simulink model "heatpump"  (R2021b)
settings: Solver=VariableStepAuto  StartTime=0.0  StopTime=10.0  RelTol=1e-3
settings Model: Creator=Sam  LastModifiedBy=Sam

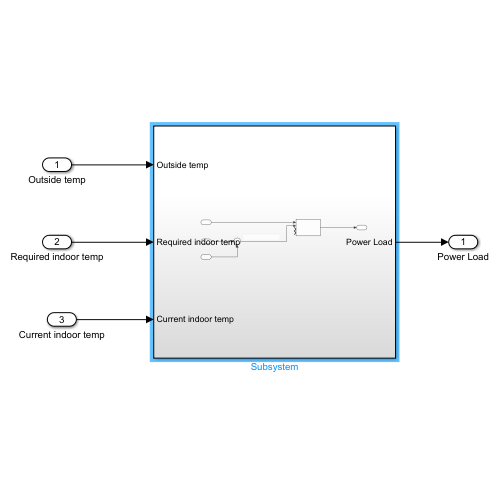
[thumbnail: Simulink's stored preview of the top-level diagram]
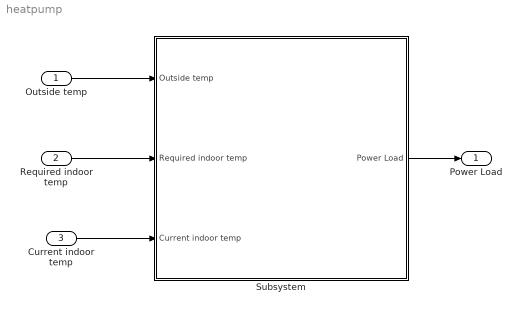
== system heatpump ==
  Outside temp : Inport
  Required indoor temp : Inport  Port=2
  Current indoor temp : Inport  Port=3
  Subsystem : Subsystem
  Power Load : Outport
  wires:
  Outside temp/1 -> Subsystem/1(Outside temp)
  Required indoor temp/1 -> Subsystem/2(Required indoor temp)
  Subsystem/1(Power Load) -> Power Load/1
  Current indoor temp/1 -> Subsystem/3(Current indoor temp)

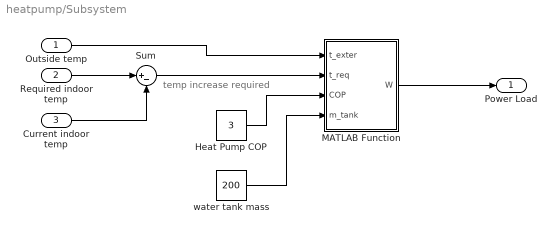
== system heatpump/Subsystem ==
  note: temp increase required
  Outside temp : Inport
  Required indoor temp : Inport  Port=2
  Current indoor temp : Inport  Port=3
  Heat Pump COP : Constant  Value=3
  MATLAB Function : MATLAB Function  TreatAsAtomicUnit=on
  Sum : Sum  Inputs=|+-
  water tank mass : Constant  Value=200
  Power Load : Outport
  wires:
  Required indoor temp/1 -> Sum/1
  Current indoor temp/1 -> Sum/2
  Outside temp/1 -> MATLAB Function/1(t_exter)
  Sum/1 -> MATLAB Function/2(t_req)
  MATLAB Function/1(W) -> Power Load/1
  water tank mass/1 -> MATLAB Function/4(m_tank)
  Heat Pump COP/1 -> MATLAB Function/3(COP)

== matlab function heatpump/Subsystem/MATLAB Function ==
  data: t_exter input; W output; t_req input; COP input; m_tank input
function W = fcn(t_exter, t_req, COP, m_tank)
%Specific heat capacity of water
c = 4182; %J/kg K

% heat extracted
Qc = m*c*(t_req - t_exter)

%Work done
W = Qc/COP;
